simulink model "adc5g_dmux_x2"  (R2012b)
settings: Solver=ode45  StartTime=0.0  StopTime=10.0  RelTol=1e-3
libraries: xbsIndex_r4 x35, dspsigops x32
settings Model: Creator=root  LastModifiedBy=root

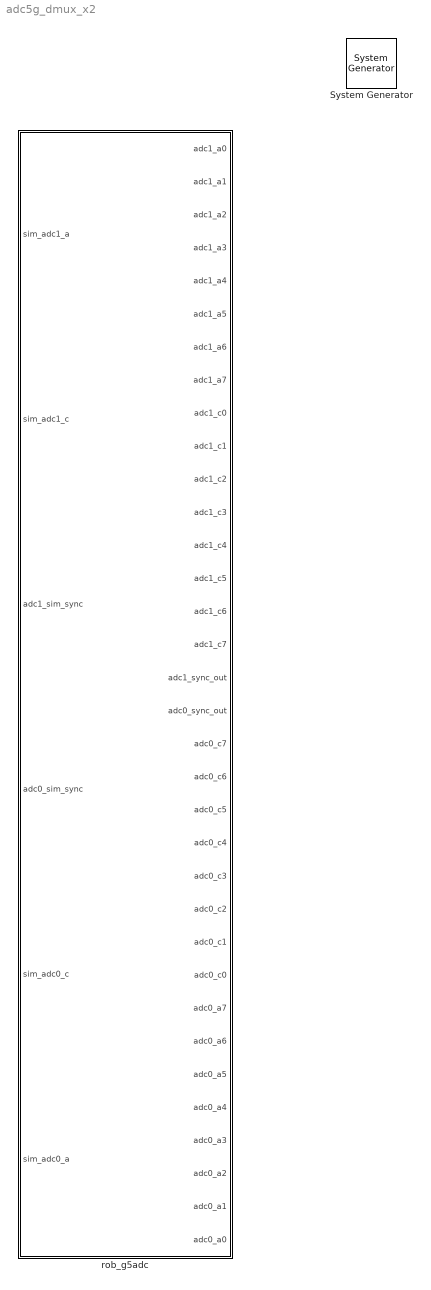
== system adc5g_dmux_x2 ==
  " System Generator" : xbsIndex_r4/ System Generator  Tag=genX  xilinxfamily=Kintex7  part=xc7k325t  speed=-3  package=fbg676  synthesis_tool=XST  clock_wrapper=Clock Enables  directory=./netlist  proj_type=Project Navigator  Synth_file=XST Defaults  Impl_file=ISE Defaults  testbench=off  simulink_period=1  sysclk_period=10  dcm_input_clock_period=10  incr_netlist=off  trim_vbits=Everywhere in SubSystem  dbl_ovrd=According to Block Masks  core_generation=According to Block Masks  run_coregen=off  deprecated_control=off  eval_field=0  block_type=sysgen
  rob_g5adc : Subsystem  Tag=xps:adc5g_dmux_x2  mask(adc5g_dmux_x2){use_adc0=on, input_mode_adc0=Two-channel -- A&C, use_adc1=on, input_mode_adc1=Two-channel -- A&C, adc_clk_rate=88, using_ctrl=on, test_ramp=off, interleave=off}
      mask prompts: use_adc0 "use ZDOK0?"; input_mode_adc0 "Input mode (ZDOK0):"; use_adc1 "use ZDOK1?"; input_mode_adc1 "Input mode (ZDOK1):"; adc_clk_rate "ADC Clock Rate (MHz):"; using_ctrl "use control"; test_ramp "start in test ramp mode"; interleave "Interleave 2 ADC boards?"
      mask help:
      | Interface for 2 of the ASIAA 5 GSps ADC. For each ZDOK? supports interleaving all four
      | cores using either input A or C, or interleaving two-cores each for
      | A and C. The hardware itself comes in two versions:
      |
      | DMUX 1:2 -- 4-bit samples, 4 parallel streams
      | DMUX 1:1 -- 8-bit samples, 2 parallel streams
      |
      | But it's only implemented for DMUX 1:1.
      |
      | I should be able to syncronise the two ADC to delete the phase delay that
      | the adc starts whit.
      mask init:
      | adc5g_dmux_x2_init(gcb,...
      |     'use_adc0', use_adc0,...
      |     'input_mode_adc0', input_mode_adc0,...
      |     'use_adc1', use_adc1,...
      |     'input_mode_adc1', input_mode_adc1,...
      |     'adc_clk_rate', adc_clk_rate,...
      |     'using_ctrl', using_ctrl,...
      |     'test_ramp', test_ramp,...
      |     'interleave', interleave);
      mask TypeOptions input_mode_adc0: One-channel -- A | One-channel -- C | Two-channel -- A&C
      mask TypeOptions input_mode_adc1: One-channel -- A | One-channel -- C | Two-channel -- A&C

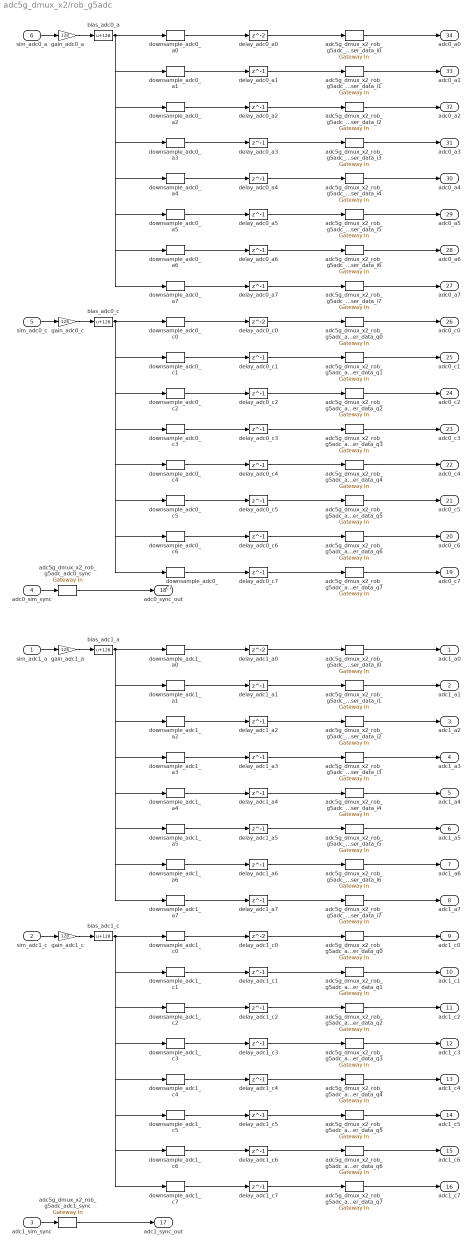
== system adc5g_dmux_x2/rob_g5adc ==
  sim_adc1_a : Inport
  sim_adc1_c : Inport  Port=2
  adc1_sim_sync : Inport  Port=3
  adc0_sim_sync : Inport  Port=4
  sim_adc0_c : Inport  Port=5
  sim_adc0_a : Inport  Port=6
  adc5g_dmux_x2_rob_g5adc_adc0_sync : xbsIndex_r4/Gateway In  gui_display_data_type=Fixed-point  arith_type=Boolean  n_bits=16  bin_pt=14  preci_type=Single  exp_width=8  frac_width=24  quantization="Round  (unbiased: +/- Inf)"  overflow=Saturate  period=1  dbl_ovrd=off  timing_constraint=None  locs_specified=off  LOCs={}  UseAsADC=off  ADCChannel='1'  inherit_from_input=off  hdl_port=on  block_type=gatewayin
  adc5g_dmux_x2_rob_g5adc_adc0_user_data_i{0..7} (8 alike) : xbsIndex_r4/Gateway In  gui_display_data_type=Fixed-point  arith_type=Unsigned  n_bits=8  bin_pt=0  preci_type=Single  exp_width=8  frac_width=24  quantization=Truncate  overflow=Wrap  period=1  dbl_ovrd=off  timing_constraint=None  locs_specified=off  LOCs={}  UseAsADC=off  ADCChannel='1'  inherit_from_input=off  hdl_port=on  block_type=gatewayin
  adc5g_dmux_x2_rob_g5adc_adc0_user_data_q{0..7} (8 alike) : xbsIndex_r4/Gateway In  gui_display_data_type=Fixed-point  arith_type=Unsigned  n_bits=8  bin_pt=0  preci_type=Single  exp_width=8  frac_width=24  quantization=Truncate  overflow=Wrap  period=1  dbl_ovrd=off  timing_constraint=None  locs_specified=off  LOCs={}  UseAsADC=off  ADCChannel='1'  inherit_from_input=off  hdl_port=on  block_type=gatewayin
  adc5g_dmux_x2_rob_g5adc_adc1_sync : xbsIndex_r4/Gateway In  gui_display_data_type=Fixed-point  arith_type=Boolean  n_bits=16  bin_pt=14  preci_type=Single  exp_width=8  frac_width=24  quantization="Round  (unbiased: +/- Inf)"  overflow=Saturate  period=1  dbl_ovrd=off  timing_constraint=None  locs_specified=off  LOCs={}  UseAsADC=off  ADCChannel='1'  inherit_from_input=off  hdl_port=on  block_type=gatewayin
  adc5g_dmux_x2_rob_g5adc_adc1_user_data_i{0..7} (8 alike) : xbsIndex_r4/Gateway In  gui_display_data_type=Fixed-point  arith_type=Unsigned  n_bits=8  bin_pt=0  preci_type=Single  exp_width=8  frac_width=24  quantization=Truncate  overflow=Wrap  period=1  dbl_ovrd=off  timing_constraint=None  locs_specified=off  LOCs={}  UseAsADC=off  ADCChannel='1'  inherit_from_input=off  hdl_port=on  block_type=gatewayin
  adc5g_dmux_x2_rob_g5adc_adc1_user_data_q{0..7} (8 alike) : xbsIndex_r4/Gateway In  gui_display_data_type=Fixed-point  arith_type=Unsigned  n_bits=8  bin_pt=0  preci_type=Single  exp_width=8  frac_width=24  quantization=Truncate  overflow=Wrap  period=1  dbl_ovrd=off  timing_constraint=None  locs_specified=off  LOCs={}  UseAsADC=off  ADCChannel='1'  inherit_from_input=off  hdl_port=on  block_type=gatewayin
  bias_adc0_a : Bias  Bias=128  SaturateOnIntegerOverflow=on
  bias_adc0_c : Bias  Bias=128  SaturateOnIntegerOverflow=on
  bias_adc1_a : Bias  Bias=128  SaturateOnIntegerOverflow=on
  bias_adc1_c : Bias  Bias=128  SaturateOnIntegerOverflow=on
  delay_adc0_a0 : Delay  InitialCondition=0  InputProcessing=Inherited
  delay_adc0_a{1..7} (7 alike) : Delay  DelayLength=1  InitialCondition=0  InputProcessing=Inherited
  delay_adc0_c0 : Delay  InitialCondition=0  InputProcessing=Inherited
  delay_adc0_c{1..7} (7 alike) : Delay  DelayLength=1  InitialCondition=0  InputProcessing=Inherited
  delay_adc1_a0 : Delay  InitialCondition=0  InputProcessing=Inherited
  delay_adc1_a{1..7} (7 alike) : Delay  DelayLength=1  InitialCondition=0  InputProcessing=Inherited
  delay_adc1_c0 : Delay  InitialCondition=0  InputProcessing=Inherited
  delay_adc1_c{1..7} (7 alike) : Delay  DelayLength=1  InitialCondition=0  InputProcessing=Inherited
  downsample_adc0_a0 : dspsigops/Downsample  N=8  phase=0  InputProcessing=Columns as channels (frame based)  RateOptions=Enforce single-rate processing  smode=Allow multirate  fmode=Maintain input frame size  ic=0
  downsample_adc0_a1 : dspsigops/Downsample  N=8  phase=1  InputProcessing=Columns as channels (frame based)  RateOptions=Enforce single-rate processing  smode=Allow multirate  fmode=Maintain input frame size  ic=0
  downsample_adc0_a2 : dspsigops/Downsample  N=8  phase=2  InputProcessing=Columns as channels (frame based)  RateOptions=Enforce single-rate processing  smode=Allow multirate  fmode=Maintain input frame size  ic=0
  downsample_adc0_a3 : dspsigops/Downsample  N=8  phase=3  InputProcessing=Columns as channels (frame based)  RateOptions=Enforce single-rate processing  smode=Allow multirate  fmode=Maintain input frame size  ic=0
  downsample_adc0_a4 : dspsigops/Downsample  N=8  phase=4  InputProcessing=Columns as channels (frame based)  RateOptions=Enforce single-rate processing  smode=Allow multirate  fmode=Maintain input frame size  ic=0
  downsample_adc0_a5 : dspsigops/Downsample  N=8  phase=5  InputProcessing=Columns as channels (frame based)  RateOptions=Enforce single-rate processing  smode=Allow multirate  fmode=Maintain input frame size  ic=0
  downsample_adc0_a6 : dspsigops/Downsample  N=8  phase=6  InputProcessing=Columns as channels (frame based)  RateOptions=Enforce single-rate processing  smode=Allow multirate  fmode=Maintain input frame size  ic=0
  downsample_adc0_a7 : dspsigops/Downsample  N=8  phase=7  InputProcessing=Columns as channels (frame based)  RateOptions=Enforce single-rate processing  smode=Allow multirate  fmode=Maintain input frame size  ic=0
  downsample_adc0_c0 : dspsigops/Downsample  N=8  phase=0  InputProcessing=Columns as channels (frame based)  RateOptions=Enforce single-rate processing  smode=Allow multirate  fmode=Maintain input frame size  ic=0
  downsample_adc0_c1 : dspsigops/Downsample  N=8  phase=1  InputProcessing=Columns as channels (frame based)  RateOptions=Enforce single-rate processing  smode=Allow multirate  fmode=Maintain input frame size  ic=0
  downsample_adc0_c2 : dspsigops/Downsample  N=8  phase=2  InputProcessing=Columns as channels (frame based)  RateOptions=Enforce single-rate processing  smode=Allow multirate  fmode=Maintain input frame size  ic=0
  downsample_adc0_c3 : dspsigops/Downsample  N=8  phase=3  InputProcessing=Columns as channels (frame based)  RateOptions=Enforce single-rate processing  smode=Allow multirate  fmode=Maintain input frame size  ic=0
  downsample_adc0_c4 : dspsigops/Downsample  N=8  phase=4  InputProcessing=Columns as channels (frame based)  RateOptions=Enforce single-rate processing  smode=Allow multirate  fmode=Maintain input frame size  ic=0
  downsample_adc0_c5 : dspsigops/Downsample  N=8  phase=5  InputProcessing=Columns as channels (frame based)  RateOptions=Enforce single-rate processing  smode=Allow multirate  fmode=Maintain input frame size  ic=0
  downsample_adc0_c6 : dspsigops/Downsample  N=8  phase=6  InputProcessing=Columns as channels (frame based)  RateOptions=Enforce single-rate processing  smode=Allow multirate  fmode=Maintain input frame size  ic=0
  downsample_adc0_c7 : dspsigops/Downsample  N=8  phase=7  InputProcessing=Columns as channels (frame based)  RateOptions=Enforce single-rate processing  smode=Allow multirate  fmode=Maintain input frame size  ic=0
  downsample_adc1_a0 : dspsigops/Downsample  N=8  phase=0  InputProcessing=Columns as channels (frame based)  RateOptions=Enforce single-rate processing  smode=Allow multirate  fmode=Maintain input frame size  ic=0
  downsample_adc1_a1 : dspsigops/Downsample  N=8  phase=1  InputProcessing=Columns as channels (frame based)  RateOptions=Enforce single-rate processing  smode=Allow multirate  fmode=Maintain input frame size  ic=0
  downsample_adc1_a2 : dspsigops/Downsample  N=8  phase=2  InputProcessing=Columns as channels (frame based)  RateOptions=Enforce single-rate processing  smode=Allow multirate  fmode=Maintain input frame size  ic=0
  downsample_adc1_a3 : dspsigops/Downsample  N=8  phase=3  InputProcessing=Columns as channels (frame based)  RateOptions=Enforce single-rate processing  smode=Allow multirate  fmode=Maintain input frame size  ic=0
  downsample_adc1_a4 : dspsigops/Downsample  N=8  phase=4  InputProcessing=Columns as channels (frame based)  RateOptions=Enforce single-rate processing  smode=Allow multirate  fmode=Maintain input frame size  ic=0
  downsample_adc1_a5 : dspsigops/Downsample  N=8  phase=5  InputProcessing=Columns as channels (frame based)  RateOptions=Enforce single-rate processing  smode=Allow multirate  fmode=Maintain input frame size  ic=0
  downsample_adc1_a6 : dspsigops/Downsample  N=8  phase=6  InputProcessing=Columns as channels (frame based)  RateOptions=Enforce single-rate processing  smode=Allow multirate  fmode=Maintain input frame size  ic=0
  downsample_adc1_a7 : dspsigops/Downsample  N=8  phase=7  InputProcessing=Columns as channels (frame based)  RateOptions=Enforce single-rate processing  smode=Allow multirate  fmode=Maintain input frame size  ic=0
  downsample_adc1_c0 : dspsigops/Downsample  N=8  phase=0  InputProcessing=Columns as channels (frame based)  RateOptions=Enforce single-rate processing  smode=Allow multirate  fmode=Maintain input frame size  ic=0
  downsample_adc1_c1 : dspsigops/Downsample  N=8  phase=1  InputProcessing=Columns as channels (frame based)  RateOptions=Enforce single-rate processing  smode=Allow multirate  fmode=Maintain input frame size  ic=0
  downsample_adc1_c2 : dspsigops/Downsample  N=8  phase=2  InputProcessing=Columns as channels (frame based)  RateOptions=Enforce single-rate processing  smode=Allow multirate  fmode=Maintain input frame size  ic=0
  downsample_adc1_c3 : dspsigops/Downsample  N=8  phase=3  InputProcessing=Columns as channels (frame based)  RateOptions=Enforce single-rate processing  smode=Allow multirate  fmode=Maintain input frame size  ic=0
  downsample_adc1_c4 : dspsigops/Downsample  N=8  phase=4  InputProcessing=Columns as channels (frame based)  RateOptions=Enforce single-rate processing  smode=Allow multirate  fmode=Maintain input frame size  ic=0
  downsample_adc1_c5 : dspsigops/Downsample  N=8  phase=5  InputProcessing=Columns as channels (frame based)  RateOptions=Enforce single-rate processing  smode=Allow multirate  fmode=Maintain input frame size  ic=0
  downsample_adc1_c6 : dspsigops/Downsample  N=8  phase=6  InputProcessing=Columns as channels (frame based)  RateOptions=Enforce single-rate processing  smode=Allow multirate  fmode=Maintain input frame size  ic=0
  downsample_adc1_c7 : dspsigops/Downsample  N=8  phase=7  InputProcessing=Columns as channels (frame based)  RateOptions=Enforce single-rate processing  smode=Allow multirate  fmode=Maintain input frame size  ic=0
  gain_adc0_a : Gain  Gain=128  SaturateOnIntegerOverflow=on  OutDataTypeStr=Inherit: Same as input  ParamDataTypeStr=Inherit: Same as input
  gain_adc0_c : Gain  Gain=128  SaturateOnIntegerOverflow=on  OutDataTypeStr=Inherit: Same as input  ParamDataTypeStr=Inherit: Same as input
  gain_adc1_a : Gain  Gain=128  SaturateOnIntegerOverflow=on  OutDataTypeStr=Inherit: Same as input  ParamDataTypeStr=Inherit: Same as input
  gain_adc1_c : Gain  Gain=128  SaturateOnIntegerOverflow=on  OutDataTypeStr=Inherit: Same as input  ParamDataTypeStr=Inherit: Same as input
  adc1_a0 : Outport
  adc1_a1 : Outport  Port=2
  adc1_a2 : Outport  Port=3
  adc1_a3 : Outport  Port=4
  adc1_a4 : Outport  Port=5
  adc1_a5 : Outport  Port=6
  adc1_a6 : Outport  Port=7
  adc1_a7 : Outport  Port=8
  adc1_c0 : Outport  Port=9
  adc1_c1 : Outport  Port=10
  adc1_c2 : Outport  Port=11
  adc1_c3 : Outport  Port=12
  adc1_c4 : Outport  Port=13
  adc1_c5 : Outport  Port=14
  adc1_c6 : Outport  Port=15
  adc1_c7 : Outport  Port=16
  adc1_sync_out : Outport  Port=17
  adc0_sync_out : Outport  Port=18
  adc0_c7 : Outport  Port=19
  adc0_c6 : Outport  Port=20
  adc0_c5 : Outport  Port=21
  adc0_c4 : Outport  Port=22
  adc0_c3 : Outport  Port=23
  adc0_c2 : Outport  Port=24
  adc0_c1 : Outport  Port=25
  adc0_c0 : Outport  Port=26
  adc0_a7 : Outport  Port=27
  adc0_a6 : Outport  Port=28
  adc0_a5 : Outport  Port=29
  adc0_a4 : Outport  Port=30
  adc0_a3 : Outport  Port=31
  adc0_a2 : Outport  Port=32
  adc0_a1 : Outport  Port=33
  adc0_a0 : Outport  Port=34
  wires:
  sim_adc0_a/1 -> gain_adc0_a/1
  sim_adc1_a/1 -> gain_adc1_a/1
  gain_adc0_a/1 -> bias_adc0_a/1
  gain_adc1_a/1 -> bias_adc1_a/1
  bias_adc0_a/1 -> downsample_adc0_a0/1, downsample_adc0_a1/1, downsample_adc0_a2/1, downsample_adc0_a3/1, downsample_adc0_a4/1, downsample_adc0_a5/1, downsample_adc0_a6/1, downsample_adc0_a7/1
  bias_adc1_a/1 -> downsample_adc1_a0/1, downsample_adc1_a1/1, downsample_adc1_a2/1, downsample_adc1_a3/1, downsample_adc1_a4/1, downsample_adc1_a5/1, downsample_adc1_a6/1, downsample_adc1_a7/1
  downsample_adc0_a0/1 -> delay_adc0_a0/1
  downsample_adc1_a0/1 -> delay_adc1_a0/1
  delay_adc0_a0/1 -> adc5g_dmux_x2_rob_g5adc_adc0_user_data_i0/1
  delay_adc1_a0/1 -> adc5g_dmux_x2_rob_g5adc_adc1_user_data_i0/1
  adc5g_dmux_x2_rob_g5adc_adc0_user_data_i0/1 -> adc0_a0/1
  adc5g_dmux_x2_rob_g5adc_adc1_user_data_i0/1 -> adc1_a0/1
  downsample_adc0_a1/1 -> delay_adc0_a1/1
  downsample_adc1_a1/1 -> delay_adc1_a1/1
  delay_adc0_a1/1 -> adc5g_dmux_x2_rob_g5adc_adc0_user_data_i1/1
  delay_adc1_a1/1 -> adc5g_dmux_x2_rob_g5adc_adc1_user_data_i1/1
  adc5g_dmux_x2_rob_g5adc_adc0_user_data_i1/1 -> adc0_a1/1
  adc5g_dmux_x2_rob_g5adc_adc1_user_data_i1/1 -> adc1_a1/1
  downsample_adc0_a2/1 -> delay_adc0_a2/1
  downsample_adc1_a2/1 -> delay_adc1_a2/1
  delay_adc0_a2/1 -> adc5g_dmux_x2_rob_g5adc_adc0_user_data_i2/1
  delay_adc1_a2/1 -> adc5g_dmux_x2_rob_g5adc_adc1_user_data_i2/1
  adc5g_dmux_x2_rob_g5adc_adc0_user_data_i2/1 -> adc0_a2/1
  adc5g_dmux_x2_rob_g5adc_adc1_user_data_i2/1 -> adc1_a2/1
  downsample_adc0_a3/1 -> delay_adc0_a3/1
  downsample_adc1_a3/1 -> delay_adc1_a3/1
  delay_adc0_a3/1 -> adc5g_dmux_x2_rob_g5adc_adc0_user_data_i3/1
  delay_adc1_a3/1 -> adc5g_dmux_x2_rob_g5adc_adc1_user_data_i3/1
  adc5g_dmux_x2_rob_g5adc_adc0_user_data_i3/1 -> adc0_a3/1
  adc5g_dmux_x2_rob_g5adc_adc1_user_data_i3/1 -> adc1_a3/1
  downsample_adc0_a4/1 -> delay_adc0_a4/1
  downsample_adc1_a4/1 -> delay_adc1_a4/1
  delay_adc0_a4/1 -> adc5g_dmux_x2_rob_g5adc_adc0_user_data_i4/1
  delay_adc1_a4/1 -> adc5g_dmux_x2_rob_g5adc_adc1_user_data_i4/1
  adc5g_dmux_x2_rob_g5adc_adc0_user_data_i4/1 -> adc0_a4/1
  adc5g_dmux_x2_rob_g5adc_adc1_user_data_i4/1 -> adc1_a4/1
  downsample_adc0_a5/1 -> delay_adc0_a5/1
  downsample_adc1_a5/1 -> delay_adc1_a5/1
  delay_adc0_a5/1 -> adc5g_dmux_x2_rob_g5adc_adc0_user_data_i5/1
  delay_adc1_a5/1 -> adc5g_dmux_x2_rob_g5adc_adc1_user_data_i5/1
  adc5g_dmux_x2_rob_g5adc_adc0_user_data_i5/1 -> adc0_a5/1
  adc5g_dmux_x2_rob_g5adc_adc1_user_data_i5/1 -> adc1_a5/1
  downsample_adc0_a6/1 -> delay_adc0_a6/1
  downsample_adc1_a6/1 -> delay_adc1_a6/1
  delay_adc0_a6/1 -> adc5g_dmux_x2_rob_g5adc_adc0_user_data_i6/1
  delay_adc1_a6/1 -> adc5g_dmux_x2_rob_g5adc_adc1_user_data_i6/1
  adc5g_dmux_x2_rob_g5adc_adc0_user_data_i6/1 -> adc0_a6/1
  adc5g_dmux_x2_rob_g5adc_adc1_user_data_i6/1 -> adc1_a6/1
  downsample_adc0_a7/1 -> delay_adc0_a7/1
  downsample_adc1_a7/1 -> delay_adc1_a7/1
  delay_adc0_a7/1 -> adc5g_dmux_x2_rob_g5adc_adc0_user_data_i7/1
  delay_adc1_a7/1 -> adc5g_dmux_x2_rob_g5adc_adc1_user_data_i7/1
  adc5g_dmux_x2_rob_g5adc_adc0_user_data_i7/1 -> adc0_a7/1
  adc5g_dmux_x2_rob_g5adc_adc1_user_data_i7/1 -> adc1_a7/1
  sim_adc0_c/1 -> gain_adc0_c/1
  sim_adc1_c/1 -> gain_adc1_c/1
  gain_adc0_c/1 -> bias_adc0_c/1
  gain_adc1_c/1 -> bias_adc1_c/1
  bias_adc0_c/1 -> downsample_adc0_c0/1, downsample_adc0_c1/1, downsample_adc0_c2/1, downsample_adc0_c3/1, downsample_adc0_c4/1, downsample_adc0_c5/1, downsample_adc0_c6/1, downsample_adc0_c7/1
  bias_adc1_c/1 -> downsample_adc1_c0/1, downsample_adc1_c1/1, downsample_adc1_c2/1, downsample_adc1_c3/1, downsample_adc1_c4/1, downsample_adc1_c5/1, downsample_adc1_c6/1, downsample_adc1_c7/1
  downsample_adc0_c0/1 -> delay_adc0_c0/1
  downsample_adc1_c0/1 -> delay_adc1_c0/1
  delay_adc0_c0/1 -> adc5g_dmux_x2_rob_g5adc_adc0_user_data_q0/1
  delay_adc1_c0/1 -> adc5g_dmux_x2_rob_g5adc_adc1_user_data_q0/1
  adc5g_dmux_x2_rob_g5adc_adc0_user_data_q0/1 -> adc0_c0/1
  adc5g_dmux_x2_rob_g5adc_adc1_user_data_q0/1 -> adc1_c0/1
  downsample_adc0_c1/1 -> delay_adc0_c1/1
  downsample_adc1_c1/1 -> delay_adc1_c1/1
  delay_adc0_c1/1 -> adc5g_dmux_x2_rob_g5adc_adc0_user_data_q1/1
  delay_adc1_c1/1 -> adc5g_dmux_x2_rob_g5adc_adc1_user_data_q1/1
  adc5g_dmux_x2_rob_g5adc_adc0_user_data_q1/1 -> adc0_c1/1
  adc5g_dmux_x2_rob_g5adc_adc1_user_data_q1/1 -> adc1_c1/1
  downsample_adc0_c2/1 -> delay_adc0_c2/1
  downsample_adc1_c2/1 -> delay_adc1_c2/1
  delay_adc0_c2/1 -> adc5g_dmux_x2_rob_g5adc_adc0_user_data_q2/1
  delay_adc1_c2/1 -> adc5g_dmux_x2_rob_g5adc_adc1_user_data_q2/1
  adc5g_dmux_x2_rob_g5adc_adc0_user_data_q2/1 -> adc0_c2/1
  adc5g_dmux_x2_rob_g5adc_adc1_user_data_q2/1 -> adc1_c2/1
  downsample_adc0_c3/1 -> delay_adc0_c3/1
  downsample_adc1_c3/1 -> delay_adc1_c3/1
  delay_adc0_c3/1 -> adc5g_dmux_x2_rob_g5adc_adc0_user_data_q3/1
  delay_adc1_c3/1 -> adc5g_dmux_x2_rob_g5adc_adc1_user_data_q3/1
  adc5g_dmux_x2_rob_g5adc_adc0_user_data_q3/1 -> adc0_c3/1
  adc5g_dmux_x2_rob_g5adc_adc1_user_data_q3/1 -> adc1_c3/1
  downsample_adc0_c4/1 -> delay_adc0_c4/1
  downsample_adc1_c4/1 -> delay_adc1_c4/1
  delay_adc0_c4/1 -> adc5g_dmux_x2_rob_g5adc_adc0_user_data_q4/1
  delay_adc1_c4/1 -> adc5g_dmux_x2_rob_g5adc_adc1_user_data_q4/1
  adc5g_dmux_x2_rob_g5adc_adc0_user_data_q4/1 -> adc0_c4/1
  adc5g_dmux_x2_rob_g5adc_adc1_user_data_q4/1 -> adc1_c4/1
  downsample_adc0_c5/1 -> delay_adc0_c5/1
  downsample_adc1_c5/1 -> delay_adc1_c5/1
  delay_adc0_c5/1 -> adc5g_dmux_x2_rob_g5adc_adc0_user_data_q5/1
  delay_adc1_c5/1 -> adc5g_dmux_x2_rob_g5adc_adc1_user_data_q5/1
  adc5g_dmux_x2_rob_g5adc_adc0_user_data_q5/1 -> adc0_c5/1
  adc5g_dmux_x2_rob_g5adc_adc1_user_data_q5/1 -> adc1_c5/1
  downsample_adc0_c6/1 -> delay_adc0_c6/1
  downsample_adc1_c6/1 -> delay_adc1_c6/1
  delay_adc0_c6/1 -> adc5g_dmux_x2_rob_g5adc_adc0_user_data_q6/1
  delay_adc1_c6/1 -> adc5g_dmux_x2_rob_g5adc_adc1_user_data_q6/1
  adc5g_dmux_x2_rob_g5adc_adc0_user_data_q6/1 -> adc0_c6/1
  adc5g_dmux_x2_rob_g5adc_adc1_user_data_q6/1 -> adc1_c6/1
  downsample_adc0_c7/1 -> delay_adc0_c7/1
  downsample_adc1_c7/1 -> delay_adc1_c7/1
  delay_adc0_c7/1 -> adc5g_dmux_x2_rob_g5adc_adc0_user_data_q7/1
  delay_adc1_c7/1 -> adc5g_dmux_x2_rob_g5adc_adc1_user_data_q7/1
  adc5g_dmux_x2_rob_g5adc_adc0_user_data_q7/1 -> adc0_c7/1
  adc5g_dmux_x2_rob_g5adc_adc1_user_data_q7/1 -> adc1_c7/1
  adc0_sim_sync/1 -> adc5g_dmux_x2_rob_g5adc_adc0_sync/1
  adc1_sim_sync/1 -> adc5g_dmux_x2_rob_g5adc_adc1_sync/1
  adc5g_dmux_x2_rob_g5adc_adc0_sync/1 -> adc0_sync_out/1
  adc5g_dmux_x2_rob_g5adc_adc1_sync/1 -> adc1_sync_out/1
